simulink model "task_6_lin"  (R2024a)
settings: Solver=VariableStepAuto  StartTime=0.0  StopTime=50  MaxStep=1e-4  RelTol=1e-4
undefined symbols (not defined in the file or in its folder): A, B, C, D, K, L, x_0
settings Model: Creator=user  LastModifiedBy=user

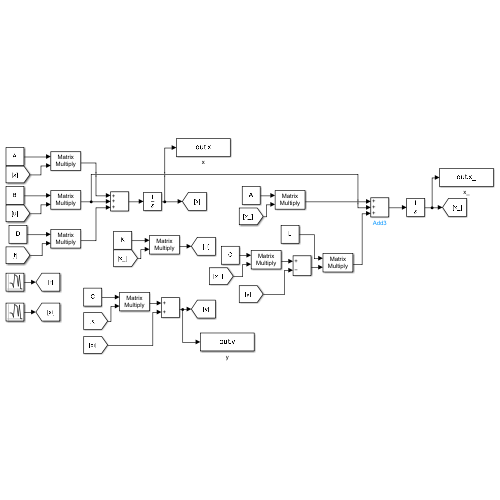
[thumbnail: Simulink's stored preview of the top-level diagram]
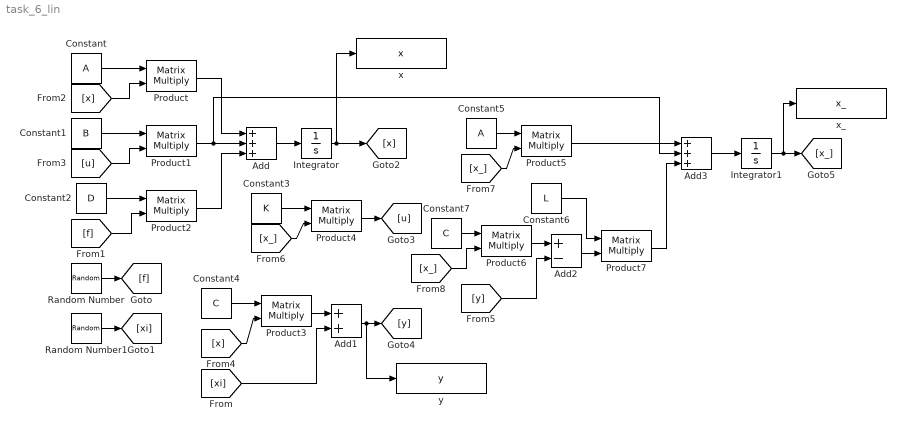
== system task_6_lin ==
  Add : Sum  Inputs=+++
  Add1 : Sum
  Add2 : Sum  Inputs=+-
  Add3 : Sum  Inputs=+++
  Constant : Constant  Value=A  VectorParams1D=off
  Constant1 : Constant  Value=B  VectorParams1D=off
  Constant2 : Constant  Value=D  VectorParams1D=off
  Constant3 : Constant  Value=K  VectorParams1D=off
  Constant4 : Constant  Value=C  VectorParams1D=off
  Constant5 : Constant  Value=A  VectorParams1D=off
  Constant6 : Constant  Value=L  VectorParams1D=off
  Constant7 : Constant  Value=C  VectorParams1D=off
  Integrator : Integrator  InitialCondition=x_0
  Integrator1 : Integrator  InitialCondition=x_0
  Product{,1..7} (8 alike) : Product  Multiplication=Matrix(*)
  Random Number : RandomNumber  Variance=0.1  Seed=[1]  SampleTime=0.001  VectorParams1D=off
  Random Number1 : RandomNumber  Variance=0.01  Seed=[2;3]  SampleTime=0.001  VectorParams1D=off
  x : ToWorkspace  VariableName=x  SaveFormat=Timeseries  SampleTime=-1
  x_ : ToWorkspace  VariableName=x_  SaveFormat=Timeseries  SampleTime=-1
  y : ToWorkspace  VariableName=y  SaveFormat=Timeseries  SampleTime=-1
  wires:
  Random Number/1 -> [f]
  Random Number1/1 -> [xi]
  Constant/1 -> Product/1
  [x] -> Product/2
  Constant1/1 -> Product1/1
  [u] -> Product1/2
  Constant2/1 -> Product2/1
  [f] -> Product2/2
  Product1/1 -> Add3/2, Add/2
  Product/1 -> Add/1
  Product2/1 -> Add/3
  Add/1 -> Integrator/1
  Constant4/1 -> Product3/1
  [x] -> Product3/2
  Product3/1 -> Add1/1
  [xi] -> Add1/2
  Add1/1 -> y/1, [y]
  Constant3/1 -> Product4/1
  [x_] -> Product4/2
  Product4/1 -> [u]
  Constant5/1 -> Product5/1
  [x_] -> Product5/2
  Constant7/1 -> Product6/1
  [x_] -> Product6/2
  Product6/1 -> Add2/1
  [y] -> Add2/2
  Add2/1 -> Product7/2
  Constant6/1 -> Product7/1
  Product5/1 -> Add3/1
  Product7/1 -> Add3/3
  Add3/1 -> Integrator1/1
  Integrator1/1 -> x_/1, [x_]
  Integrator/1 -> x/1, [x]
